simulink model "camshaft_valve"  (R2023a)
settings: Solver=FixedStepAuto  StartTime=0.0  StopTime=3  FixedStep=0.0001  RelTol=1e-3
libraries: dspstat3 x1
settings Model: Creator=saidb  LastModifiedBy=saidb

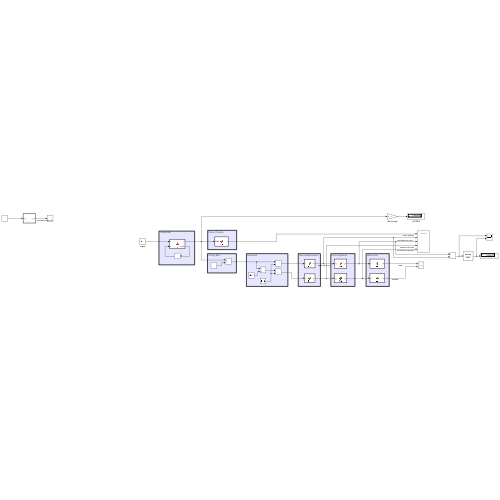
[thumbnail: Simulink's stored preview of the top-level diagram]
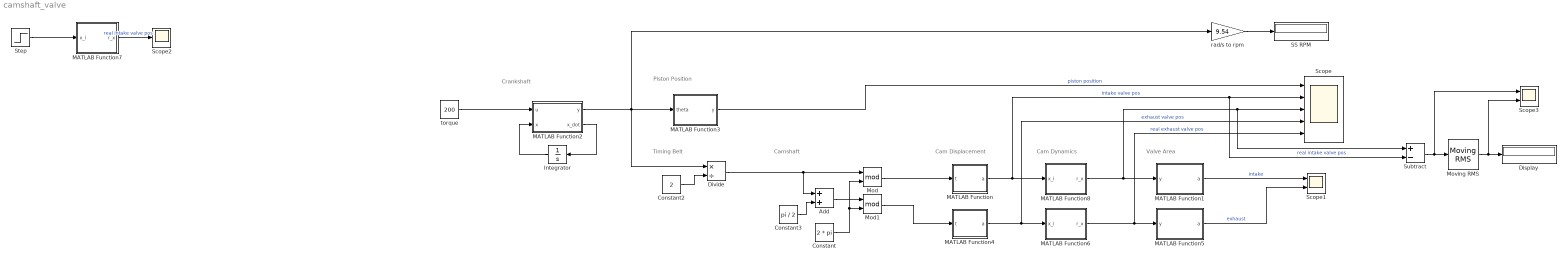
== system camshaft_valve ==
  note: Cam Dynamics
  note: Camshaft
  note: Valve Area
  note: Cam Displacement
  note: Piston Position
  note: Timing Belt
  note: Crankshaft
  Add : Sum
  Constant : Constant  Value=2 * pi
  Constant2 : Constant  Value=2
  Constant3 : Constant  Value=pi / 2
  Display : Display
  Divide : Product  Inputs=*/
  Integrator : Integrator  InitialCondition=[0;0]
  MATLAB Function : MATLAB Function  TreatAsAtomicUnit=on
  MATLAB Function1 : MATLAB Function  TreatAsAtomicUnit=on
  MATLAB Function2 : MATLAB Function  TreatAsAtomicUnit=on
  MATLAB Function3 : MATLAB Function  TreatAsAtomicUnit=on
  MATLAB Function4 : MATLAB Function  TreatAsAtomicUnit=on
  MATLAB Function5 : MATLAB Function  TreatAsAtomicUnit=on
  MATLAB Function6 : MATLAB Function  TreatAsAtomicUnit=on
  MATLAB Function7 : MATLAB Function  TreatAsAtomicUnit=on
  MATLAB Function8 : MATLAB Function  TreatAsAtomicUnit=on
  Mod : Math  Operator=mod
  Mod1 : Math  Operator=mod
  Moving RMS : dspstat3/Moving RMS  Method=Sliding window  ForgettingFactorPort=off  SpecifyWindowLength=on  WindowLength=4  OverlapLength=3  AllowArbitraryInputLength=off  ForgettingFactor=0.9  SimulateUsing=Code generation
  SS RPM : Display
  Scope : Scope  NumInputPorts=5
  Scope1 : Scope  NumInputPorts=2
  Scope2 : Scope
  Scope3 : Scope  NumInputPorts=2
  Step : Step  Before=0.01  After=-5  SampleTime=0
  Subtract : Sum  Inputs=+-
  rad/s to rpm : Gain  Gain=9.54
  torque : Constant  Value=200
  wires:
  Constant/1 -> Mod/2, Mod1/2
  Mod/1 -> MATLAB Function/1(t)
  MATLAB Function1/1(a) -> Scope1/1  "intake"
  MATLAB Function2/2(x_dot) -> Integrator/1
  Integrator/1 -> MATLAB Function2/2(x)
  torque/1 -> MATLAB Function2/1(u)
  Constant2/1 -> Divide/2
  MATLAB Function/1(a) -> Subtract/2, Scope/2, MATLAB Function8/1(x_i)  "intake valve pos"
  MATLAB Function3/1(y) -> Scope/1  "piston position"
  MATLAB Function2/1(y) -> rad/s to rpm/1, Divide/1, MATLAB Function3/1(theta)
  Divide/1 -> Add/1, Mod/1
  Mod1/1 -> MATLAB Function4/1(t)
  Add/1 -> Mod1/1
  Constant3/1 -> Add/2
  MATLAB Function4/1(a) -> Scope/4, MATLAB Function6/1(x_i)  "exhaust valve pos"
  MATLAB Function5/1(a) -> Scope1/2  "exhaust"
  MATLAB Function8/1(r_x) -> Subtract/1, Scope/3, MATLAB Function1/1(y)  "real intake valve pos"
  MATLAB Function6/1(r_x) -> Scope/5, MATLAB Function5/1(y)  "real exhaust valve pos"
  rad/s to rpm/1 -> SS RPM/1
  Step/1 -> MATLAB Function7/1(x_i)
  MATLAB Function7/1(r_x) -> Scope2/1  "real intake valve pos"
  Subtract/1 -> Scope3/1, Moving RMS/1
  Moving RMS/1 -> Scope3/2, Display/1

== matlab function camshaft_valve/MATLAB Function1 ==
  data: y input; a output
function a = fcn(y)

pi = 3.141592;
r = 0.02;

a = 2 * pi * r * y;

if a >= pi * r^2
    a = pi * r^2;
end

end

== matlab function camshaft_valve/MATLAB Function ==
  data: t input; a output
function a = fcn(t)

e = 2.71828;
pi = 3.141592;
r = 0.02;

maxInputArea = pi * r^2;

maxValveDisplacement = maxInputArea / (2 * pi * r);

a = (e^(-((2 * t) - (pi / 2))^4) * maxValveDisplacement) + 0.01;

end

== matlab function camshaft_valve/MATLAB Function2 ==
  data: y output; u input; x input; x_dot output
function [y, x_dot] = fcn(u, x)

I = 0.19215;
c = 0.32236;
k = 0;

A = [  0     1  ;
     -k/I  -c/I];
B = [ 0  ;
     1/I];
C = [1 0];
D = 0;

x_dot = A * x + B * u;
y = C * x + D * u;

== matlab function camshaft_valve/MATLAB Function3 ==
  data: theta input; y output
function y  = fcn(theta)

l1 = 0.05;
l2 = 0.1;
e = 0;
h = 0;

y = sqrt(l2^2 - (l1 * sin(theta) + e)^2) + l1 * cos(theta) + h;

== matlab function camshaft_valve/MATLAB Function4 ==
  data: t input; a output
function a = fcn(t)

e = 2.71828;
pi = 3.141592;
r = 0.02;

maxInputArea = pi * r^2;

maxValveDisplacement = maxInputArea / (2 * pi * r);

a = e^(-((2 * t) - (pi / 2))^4) * maxValveDisplacement;

end

== matlab function camshaft_valve/MATLAB Function5 ==
  data: y input; a output
function a = fcn(y)

pi = 3.141592;
r = 0.02;

a = 2 * pi * r * y;

if a >= pi * r^2
    a = pi * r^2;
end

end

== matlab function camshaft_valve/MATLAB Function6 ==
  settings: updateMethod=DISCRETE
  data: r_x output; x_i input
function r_x = fcn(x_i)

dt = 0.0001;
preload = 0;

persistent x
persistent x_dot
persistent x_i_l;

if isempty(x_i_l)
    x_i_l = preload;
end

x_i_d = (x_i - x_i_l) / dt;

if isempty(x_dot)
    x_dot = [0 ; 0];
end
if isempty(x)
    x = [preload ; 0];
else
    x_temp = x + x_dot * dt;
    if x_temp(1) < x_i
        x(1) = x_i;
        x(2) = x_i_d - (x(2) - x_i_d) * 0.5;
    else
        x = x + x_dot * dt;
    end
end

m = 0.1 + 0.1;
c = 100;
k = 65000;
A = [  0     1  ;
     -k/m  -c/m];

x_dot = A * x;

x_i_l = x_i;
r_x = x(1);

== matlab function camshaft_valve/MATLAB Function7 ==
  settings: updateMethod=DISCRETE
  data: r_x output; x_i input
function r_x = fcn(x_i)

dt = 0.0001;

persistent x
persistent x_dot
persistent x_i_l;

if isempty(x_i_l)
    x_i_l = 0.01;
end

x_i = x_i + 0.01;

x_i_d = (x_i - x_i_l) / dt;

if isempty(x_dot)
    x_dot = [0 ; 0];
end
if isempty(x)
    x = [0.01 ; 0];
else
    x_temp = x + x_dot * dt;
    if x_temp(1) < x_i
        x(1) = x_i;
        x(2) = x_i_d - (x(2) - x_i_d);
    else
        x = x + x_dot * dt;
    end
end

m = 0.1 + 0.1;
c = 100;
k = 65000;
A = [  0     1  ;
     -k/m  -c/m];

x_dot = A * x;

x_i_l = x_i;
r_x = x(1);

== matlab function camshaft_valve/MATLAB Function8 ==
  settings: updateMethod=DISCRETE
  data: r_x output; x_i input
function r_x = fcn(x_i)

dt = 0.0001;
preload = 0.01;

persistent x
persistent x_dot
persistent x_i_l;

if isempty(x_i_l)
    x_i_l = preload;
end

x_i_d = (x_i - x_i_l) / dt;

if isempty(x_dot)
    x_dot = [0 ; 0];
end
if isempty(x)
    x = [preload ; 0];
else
    x_temp = x + x_dot * dt;
    if x_temp(1) < x_i
        x(1) = x_i;
        x(2) = x_i_d - (x(2) - x_i_d) * 0.5;
    else
        x = x + x_dot * dt;
    end
end

m = 0.1 + 0.1;
c = 100;
k = 120000;
A = [  0     1  ;
     -k/m  -c/m];

x_dot = A * x;

x_i_l = x_i;
r_x = x(1);
